simulink model "OneWheelModel_3"  (R2021b)
settings: Solver=ode4  StartTime=0.0  StopTime=1  FixedStep=0.001  RelTol=1e-3
values from neighbouring files (symbols this model uses):
  afx_f = [1.736519934348130,-2.903281841026900e-04,2.651682004580759,7.000047010028531e+04,3.270011055825476e+03,-0.001252141095807,1.596836353939939]    [OneWheelModel_test1.m]    (also in OneWheelModel_test2.m)
  Iwf = 0.2    [OneWheelModel_test1.m]    (also in OneWheelModel_test2.m)
  M = 260    [OneWheelModel_test1.m]    (also in OneWheelModel_test2.m)
  mu_tire_F = 0.55    [OneWheelModel_test1.m]    (also in OneWheelModel_test2.m)
  Rwf = 18*(25.4/1000)/2    (= 0.2286)    [OneWheelModel_test1.m]    (also in OneWheelModel_test2.m)
undefined symbols (not defined in the file or in its folder): g, gear_f, Mwf, W0_R
settings Model: Creator=tsuyoshi  LastModifiedBy=tsuyoshi

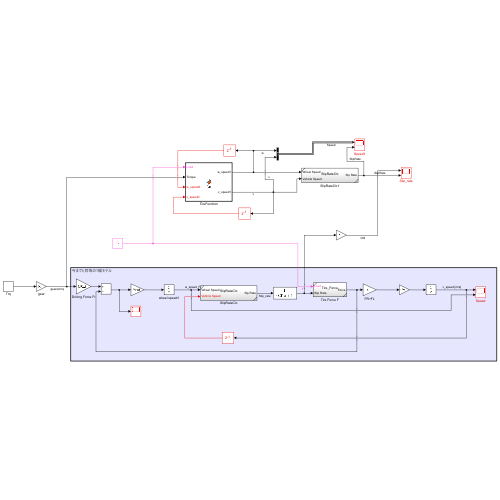
[thumbnail: Simulink's stored preview of the top-level diagram]
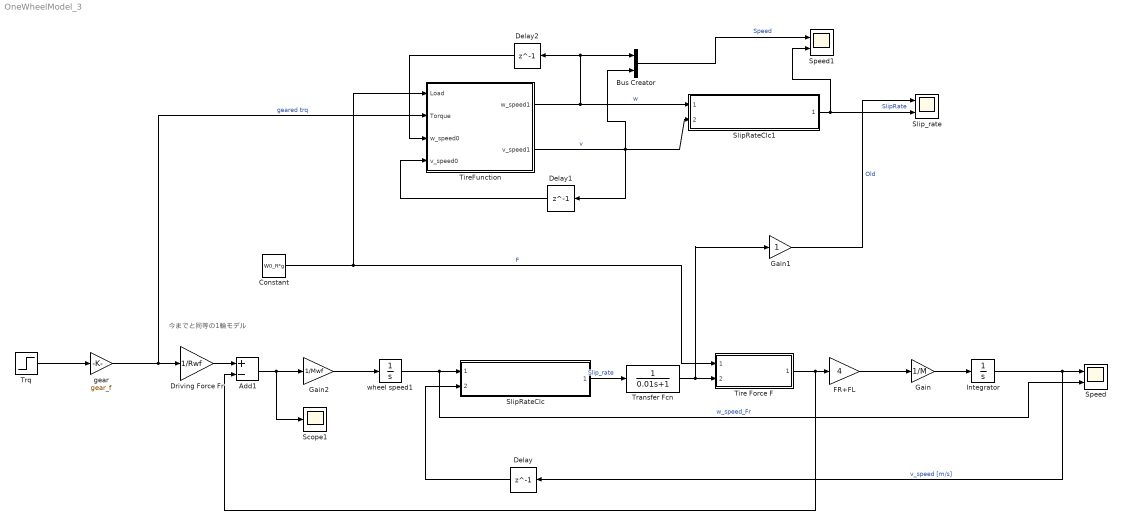
== system OneWheelModel_3 ==
  note: 今までと同等の1輪モデル
  Add1 : Sum  Inputs=+-
  Bus Creator : BusCreator  Inputs=2
  Constant : Constant  Value=W0_R*g
  Delay : Delay  DelayLength=1
  Delay1 : Delay  DelayLength=1
  Delay2 : Delay  DelayLength=1
  Driving Force Fr : Gain  Gain=1/Rwf
  FR+FL : Gain  Gain=4
  Gain : Gain  Gain=1/M
  Gain1 : Gain
  Gain2 : Gain  Gain=1/Mwf
  Integrator : Integrator
  Scope1 : Scope
  SlipRateClc : Subsystem  ReferencedSubsystem=SlipRateClc
  SlipRateClc1 : Subsystem  ReferencedSubsystem=SlipRateClc
  Slip_rate : Scope  NumInputPorts=2
  Speed : Scope  NumInputPorts=2
  Speed1 : Scope  NumInputPorts=2
  Tire Force F : Subsystem  ReferencedSubsystem=Tire_Force
  TireFunction : MATLAB Function  TreatAsAtomicUnit=on
  Transfer Fcn : TransferFcn  Denominator=[0.01 1]
  Trq : Step  Time=0.2  After=13  SampleTime=0
  gear : Gain  Gain=gear_f
  wheel speed1 : Integrator  LowerSaturationLimit=0
  wires:
  SlipRateClc/1 -> Transfer Fcn/1  "Slip_rate"
  Driving Force Fr/1 -> Add1/1
  Constant/1 -> Tire Force F/1, TireFunction/1(Load)  "F"
  Integrator/1 -> Speed/1, Delay/1  "v_speed [m/s]"
  Tire Force F/1 -> FR+FL/1, Add1/2
  wheel speed1/1 -> Speed/2, SlipRateClc/1  "w_speed_Fr"
  Gain/1 -> Integrator/1
  Trq/1 -> gear/1
  gear/1 -> TireFunction/2(Torque), Driving Force Fr/1  "geared trq"
  FR+FL/1 -> Gain/1
  Gain2/1 -> wheel speed1/1
  Add1/1 -> Gain2/1, Scope1/1
  Delay/1 -> SlipRateClc/2
  TireFunction/1(w_speed1) -> SlipRateClc1/1, Bus Creator/1, Delay2/1  "w"
  TireFunction/2(v_speed1) -> Bus Creator/2, Delay1/1, SlipRateClc1/2  "v"
  SlipRateClc1/1 -> Speed1/2, Slip_rate/2  "SlipRate"
  Delay1/1 -> TireFunction/4(v_speed0)
  Delay2/1 -> TireFunction/3(w_speed0)
  Gain1/1 -> Slip_rate/1  "Old"
  Bus Creator/1 -> Speed1/1  "Speed"
  Transfer Fcn/1 -> Gain1/1, Tire Force F/2

== matlab function OneWheelModel_3/TireFunction ==
  data: Load input; Torque input; w_speed0 input; v_speed0 input; w_speed1 output; Rwf parameter; Iwf parameter; afx_f parameter; mu_tire_F parameter; v_speed1 output; M parameter
function [w_speed1, v_speed1] = fcn(Load, Torque, w_speed0, v_speed0, Rwf, Iwf, afx_f, mu_tire_F, M)
%%
% Input
% v_speed0 : vehicle speed [m/s]
% w_speed0 : wheel speed [m/s]

%% main
TimeStep=0.001;

if w_speed0==0
    if Torque>0
        %w_speed0=Rwf*Torque/Iwf * TimeStep;
        w_speed0=0.1;
    else
        w_speed1=0;
        v_speed1=0;
        return
    end
end
    
    x0=[w_speed0; v_speed0];
    [t,x] = ode45(@myfun,[0 TimeStep],x0);
    w_speed1=x(length(t),1);
    v_speed1=x(length(t),2);

    function dxdt=myfun(t,x)
        w_speed=x(1);
        v_speed=x(2);
        lambda=(w_speed-v_speed)/w_speed;
        C = afx_f(1);
        D = (Load*afx_f(2) + afx_f(3))*Load;
        E = Load*afx_f(6) + afx_f(7);
        B = afx_f(4)*sin(2*atan(Load/afx_f(5)))/(D*C);
        F = D*sin(C*atan(B*lambda-E*(B*lambda-atan(B*lambda))))*mu_tire_F;
        w_speed_dot=Rwf/Iwf*(Torque - Rwf*F);
        v_speed_dot=4*F/M;
        dxdt=[w_speed_dot; v_speed_dot];
    end
end



% function lambda=SlipRate(w_speed, v_speed)
%     lambda=(w_speed-v_speed)/w_speed;
% %     lambda=(w_speed-v_speed)/max(w_speed,v_speed,eps);
% %     if lambda>1 
% %         lambda=1;
% %     elseif lambda<0
% %         lambda=0;
% %     end
% end
